simulink model "rate_limiter_lowpass_compensator"  (R2015b)
settings: Solver=VariableStepAuto  StartTime=0.0  StopTime=100.0  FixedStep=1e-3  MaxStep=1e-3  MinStep=1e-5  RelTol=1e-6
settings Model: Creator=dell  LastModifiedBy=dell

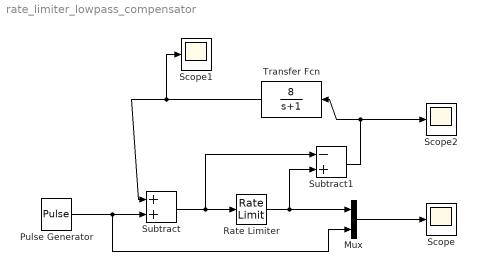
== system rate_limiter_lowpass_compensator ==
  Mux : Mux  Inputs=2
  Pulse Generator : DiscretePulseGenerator  PulseType=Time based  Period=10  PulseWidth=40
  Rate Limiter : RateLimiter  SampleTimeMode=inherited
  Scope : Scope
  Scope1 : Scope
  Scope2 : Scope
  Subtract : Sum
  Subtract1 : Sum  Inputs=-+
  Transfer Fcn : TransferFcn  Numerator=[8]  Denominator=[1 1]
  wires:
  Subtract/1 -> Subtract1/1, Rate Limiter/1
  Rate Limiter/1 -> Mux/1, Subtract1/2
  Subtract1/1 -> Scope2/1, Transfer Fcn/1
  Transfer Fcn/1 -> Scope1/1, Subtract/1
  Pulse Generator/1 -> Mux/2, Subtract/2
  Mux/1 -> Scope/1
